simulink model "mcb_pmsm_param_est_f28379d"  (R2024b)
settings: Solver=FixedStepDiscrete  StartTime=0.0  StopTime=12  RelTol=1e-3  EnableMultiTasking=on
InitFcn:
  | mcb_pmsm_param_est_f28379d_data;
values from neighbouring files (symbols this model uses):
  dataType = 'single'    [mcb_pmsm_param_est_f28379d_data.m]
  inverter = evalin('base','inverter')    [mcb_param_est_StopFunc.m]    (also in mcb_pmsm_param_est_f28379d_data.m = mcb_updateInverterParameters(motor,inverter,target))
  target = mcb_SetProcessorDetails('F28379D',PWM_frequency)    [mcb_pmsm_param_est_f28379d_data.m]
  Ts = T_pwm    (= 5e-05)    [mcb_pmsm_param_est_f28379d_data.m]
  Ts_motor = T_pwm/2    (= 2.5e-05)    [mcb_pmsm_param_est_f28379d_data.m]
undefined symbols (not defined in the file or in its folder): Down, GPTRIP1SEL, GPTRIP2SEL, motor, TZ1, TZ2, Up
libraries: simulink x14, c2802xlib x8, c280xlib x5, mcbpmsmparamestlib x5, c2837xDlib x4, mcbpositiondecoderlib x3, svdschedulerlib x2, autolibpmsminterior x2, mcbplantlib x1, mcbcontrolslib x1, svdutilitieslib x1
(part 1 of 3)
settings Model: DataDictionary=mcbEnumerations.sldd  ExtModeTrigDuration=8  Creator=The MathWorks, Inc.  LastModifiedBy=The MathWorks, Inc.
settings SolverCC: AlgebraicLoopSolver=TrustRegion
settings OptimizationCC: DefaultParameterBehavior=Inlined  DefaultUnderspecifiedDataType=single  OptimizeBlockIOStorage=off  ReuseModelBlockBuffer=off  EnhancedBackFolding=on  InitFltsAndDblsToZero=on  NoFixptDivByZeroProtection=on  EfficientFloat2IntCast=on  EfficientMapNaN2IntZero=off  MaxStackSize=1024  OptimizeBlockOrder=speed  DifferentSizesBufferReuse=on  DenormalBehavior=FlushToZero  EfficientTunableParamExpr=on
settings DebuggingCC: MultiTaskDSMMsg=none  ParameterPrecisionLossMsg=none  ParameterTunabilityLossMsg=error  UnconnectedInputMsg=warning  UnconnectedOutputMsg=warning  UnconnectedLineMsg=warning  SubsystemReferenceDiagnosticForUnitTest=warning
settings HardwareCC: ProdBitPerChar=16  ProdBitPerInt=16  ProdBitPerPointer=32  ProdBitPerSizeT=32  ProdBitPerPtrDiffT=32  ProdLargestAtomicInteger=Integer  ProdLargestAtomicFloat=None  ProdWordSize=16  ProdLongLongMode=on  ProdHWDeviceType=Texas Instruments->C2000
settings ModelReferenceCC: EnableRefExpFcnMdlSchedulingChecks=on
settings SFSimCC: MATLABDynamicMemAlloc=off
settings RTWCC: Description=Embedded Coder  SystemTargetFile=ert.tlc  HardwareBoard=TI Delfino F28379D LaunchPad  TemplateMakefile=ert_default_tmf  GenerateReport=on  Toolchain=Texas Instruments Code Composer Studio (C2000)  GPUComputeCapability=3.5  DLArmComputeVersion=19.05
settings CodeAppCC: IgnoreCustomStorageClasses=off  StateflowObjectComments=on
settings ERTTargetCC: CodeReplacementLibrary=TI C28x  ExtModeStaticAllocSize=10000  InlinedParameterPlacement=Hierarchical  ConvertIfToSwitch=off  SuppressUnreachableDefaultCases=off  MemSecPackage=tic2000demospkg  DynamicArrayContainerType=coder::array

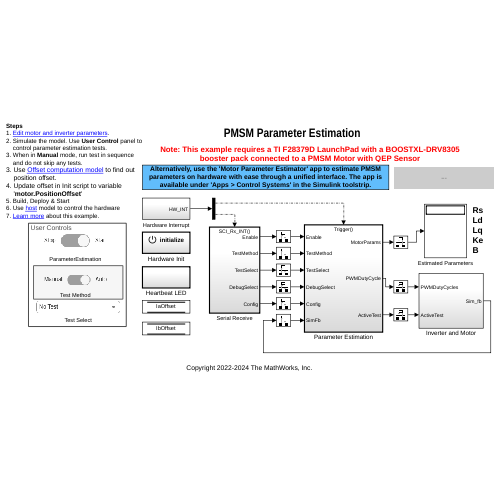
[thumbnail: Simulink's stored preview of the top-level diagram]
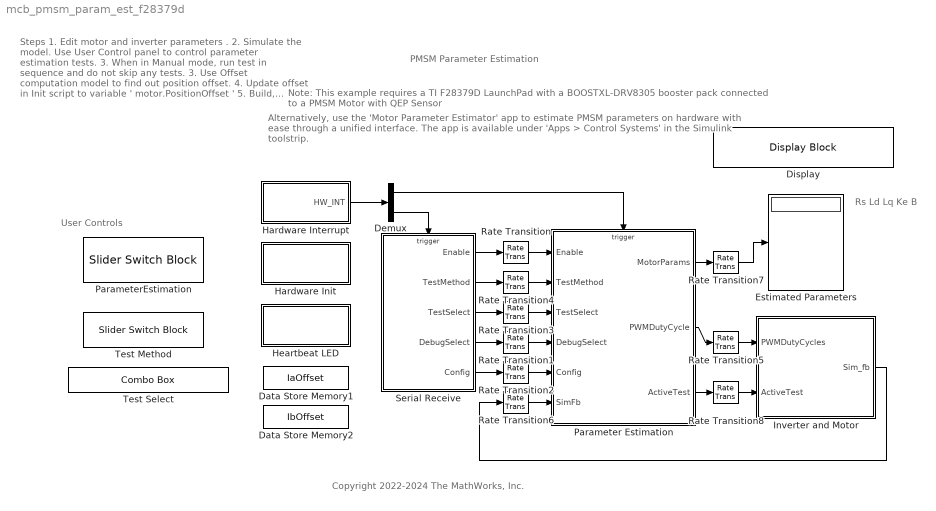
== system mcb_pmsm_param_est_f28379d ==
  note: Alternatively, use the 'Motor Parameter Estimator' app to estimate PMSM parameters on hardware with ease through a unified interface. The app is available under 'Apps > Control Systems' in the Simulink toolstrip.
  note: Note: This example requires a TI F28379D LaunchPad with a BOOSTXL-DRV8305 booster pack connected to a PMSM Motor with QEP Sensor
  note: Copyright 2022-2024 The MathWorks, Inc.
  note: PMSM Parameter Estimation
  note: Rs
      | Ld
      | Lq
      | Ke
      | B
  note: User Controls
  note: Steps
      | 1. Edit motor and inverter parameters .
      | 2. Simulate the model. Use User Control panel to
      | control parameter estimation tests.
      | 3. When in Manual mode, run test in sequence
      | and do not skip any tests.
      | 3. Use Offset computation model to find out
      | position offset.
      | 4. Update offset in Init script to variable
      | ' motor.PositionOffset '
      | 5. Build, Deploy & Start
      | 6. Use host model to control the hardware
      | 7. Learn more about this example.
  Data Store Memory1 : DataStoreMemory  DataStoreName=IaOffset  ReadBeforeWriteMsg=warning  WriteAfterWriteMsg=warning  WriteAfterReadMsg=warning  InitialValue=inverter.CtSensAOffset  ShowAdditionalParam=off
  Data Store Memory2 : DataStoreMemory  DataStoreName=IbOffset  ReadBeforeWriteMsg=warning  WriteAfterWriteMsg=warning  WriteAfterReadMsg=warning  InitialValue=inverter.CtSensBOffset  ShowAdditionalParam=off
  Demux : Demux  Outputs=2
  Display : DisplayBlock  LabelPosition=Hide  Transparency=1
  Estimated Parameters : Display
  Hardware Init : Subsystem  TreatAsAtomicUnit=on
  Hardware Interrupt : Subsystem
  Heartbeat LED : Subsystem  TreatAsAtomicUnit=on
  Inverter and Motor : Subsystem
  Parameter Estimation : Subsystem
  ParameterEstimation : SliderSwitchBlock  LabelPosition=Hide
      settings: Values={{'Stop', 'Start'}, [0 1]}
  Rate Transition{,1..6,8} (8 alike) : RateTransition  Deterministic=off
  Rate Transition7 : RateTransition  Deterministic=off  OutPortSampleTime=0.1
  Serial Receive : Subsystem  SystemSampleTime=1e-3
  Test Method : SliderSwitchBlock  LabelPosition=Hide
      settings: Values={{'Manual', 'Auto'}, [0 1]}
  Test Select : ComboBox  LabelPosition=Hide  SelectedLabel=No Test
      settings: Values={{'No Test', 'Rs', 'Ld', 'Lq', 'Ke, J, B'}, [0 1 2 3 4]}
  wires:
  Demux/1 -> Parameter Estimation/Trigger
  Demux/2 -> Serial Receive/Trigger
  Serial Receive/1(Enable) -> Rate Transition/1
  Rate Transition/1 -> Parameter Estimation/1(Enable)
  Serial Receive/5(Config) -> Rate Transition2/1
  Rate Transition2/1 -> Parameter Estimation/5(Config)
  Serial Receive/3(TestSelect) -> Rate Transition3/1
  Rate Transition3/1 -> Parameter Estimation/3(TestSelect)
  Rate Transition4/1 -> Parameter Estimation/2(TestMethod)
  Serial Receive/2(TestMethod) -> Rate Transition4/1
  Inverter and Motor/1(Sim_fb) -> Rate Transition6/1
  Parameter Estimation/2(PWMDutyCycle) -> Rate Transition5/1
  Rate Transition5/1 -> Inverter and Motor/1(PWMDutyCycles)
  Rate Transition6/1 -> Parameter Estimation/6(SimFb)
  Parameter Estimation/1(MotorParams) -> Rate Transition7/1
  Rate Transition7/1 -> Estimated Parameters/1
  Hardware Interrupt/1(HW_INT) -> Demux/1
  Serial Receive/4(DebugSelect) -> Rate Transition1/1
  Rate Transition1/1 -> Parameter Estimation/4(DebugSelect)
  Parameter Estimation/3(ActiveTest) -> Rate Transition8/1
  Rate Transition8/1 -> Inverter and Motor/2(ActiveTest)

== system mcb_pmsm_param_est_f28379d/Hardware Init ==
  6PWM_Mode : Constant  Priority=1000  Value=0x3A16  OutDataTypeStr=uint16  SampleTime=-1
  ADC_Gain_Setting : Constant  Priority=1000  Value=inverter.SPI_Gain_Setting  OutDataTypeStr=uint16  SampleTime=-1
  Event Listener : EventListener  DisableCoverage=on  EventName=reset
  Mux : Mux  Inputs=2
  Variant Subsystem : Subsystem  Variant=on  VariantControlMode=sim codegen switching
  wires:
  6PWM_Mode/1 -> Mux/1
  ADC_Gain_Setting/1 -> Mux/2
  Mux/1 -> Variant Subsystem/1(In1)

== system mcb_pmsm_param_est_f28379d/Hardware Interrupt ==
  Hardware Interrupt : Subsystem  Variant=on  VariantControlMode=sim codegen switching
  HW_INT : Outport
  wires:
  Hardware Interrupt/1(HW_INT) -> HW_INT/1

== system mcb_pmsm_param_est_f28379d/Heartbeat LED ==
  note: Heartbeat LED 1HZ
  Heartbeat LED : Subsystem  Variant=on  VariantControlMode=sim codegen switching
  RED_LED : Constant  OutDataTypeStr=uint16  SampleTime=0.5
  wires:
  RED_LED/1 -> Heartbeat LED/1(In1)

== system mcb_pmsm_param_est_f28379d/Inverter and Motor ==
  PWMDutyCycles : Inport
  ActiveTest : Inport  Port=2
  Inverter and Motor : Subsystem  Variant=on  VariantControlMode=sim codegen switching
  Sim_fb : Outport  VectorParamsAs1DForOutWhenUnconnected=off
  wires:
  PWMDutyCycles/1 -> Inverter and Motor/1(DutyCycles)
  Inverter and Motor/1(SimFb) -> Sim_fb/1
  ActiveTest/1 -> Inverter and Motor/2(ActiveTest)

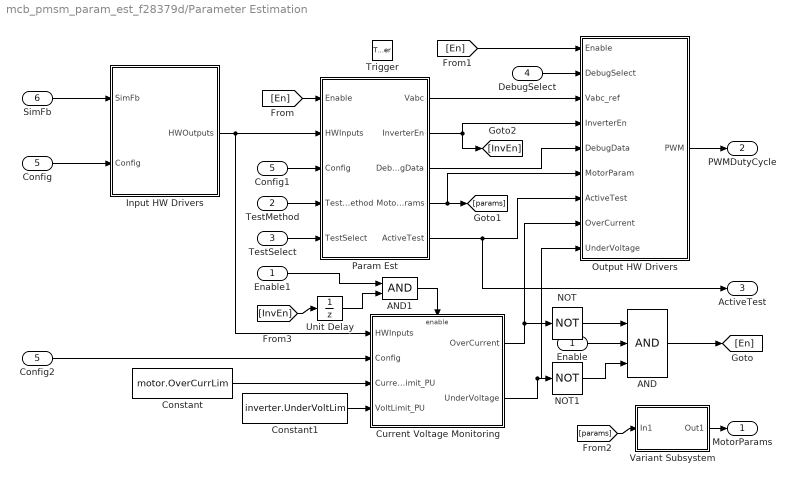
== system mcb_pmsm_param_est_f28379d/Parameter Estimation ==
  Enable : Inport
  TestMethod : Inport  Port=2
  TestSelect : Inport  Port=3
  DebugSelect : Inport  Port=4
  Config : Inport  Port=5
  SimFb : Inport  Port=6
  Trigger : TriggerPort  TriggerType=function-call  VariantControl=Variant  PortDimensions=1
  AND : Logic  Inputs=3  IconShape=distinctive  AllPortsSameDT=off  OutDataTypeStr=boolean
  AND1 : Logic  AllPortsSameDT=off  OutDataTypeStr=boolean
  Config1 : InportShadow  Port=5
  Config2 : InportShadow  Port=5
  Constant : Constant  Value=motor.OverCurrLim  OutDataTypeStr=dataType
  Constant1 : Constant  Value=inverter.UnderVoltLim  OutDataTypeStr=dataType
  Current Voltage Monitoring : Subsystem
  Enable1 : InportShadow
  Input HW Drivers : Subsystem
  NOT : Logic  Operator=NOT  IconShape=distinctive  AllPortsSameDT=off  OutDataTypeStr=boolean
  NOT1 : Logic  Operator=NOT  IconShape=distinctive  AllPortsSameDT=off  OutDataTypeStr=boolean
  Output HW Drivers : Subsystem
  Param Est : Subsystem
  Unit Delay : UnitDelay  SampleTime=-1  HasFrameUpgradeWarning=on
  Variant Subsystem : Subsystem  Variant=on  VariantControlMode=sim codegen switching
  MotorParams : Outport
  PWMDutyCycle : Outport  Port=2
  ActiveTest : Outport  Port=3
  wires:
  Config/1 -> Input HW Drivers/2(Config)
  Param Est/1(Vabc) -> Output HW Drivers/3(Vabc_ref)
  Param Est/2(InverterEn) -> Output HW Drivers/4(InverterEn), [InvEn]
  Param Est/4(MotorParams) -> Output HW Drivers/6(MotorParam), [params]
  Input HW Drivers/1(HWOutputs) -> Param Est/2(HWInputs), Current Voltage Monitoring/1(HWInputs)
  TestSelect/1 -> Param Est/5(TestSelect)
  TestMethod/1 -> Param Est/4(TestMethod)
  SimFb/1 -> Input HW Drivers/1(SimFb)
  Output HW Drivers/1(PWM) -> PWMDutyCycle/1
  Variant Subsystem/1(Out1) -> MotorParams/1
  [En] -> Output HW Drivers/1(Enable)
  Config1/1 -> Param Est/3(Config)
  Config2/1 -> Current Voltage Monitoring/2(Config)
  Param Est/3(DebugData) -> Output HW Drivers/5(DebugData)
  DebugSelect/1 -> Output HW Drivers/2(DebugSelect)
  Constant/1 -> Current Voltage Monitoring/3(CurrentLimit_PU)
  Constant1/1 -> Current Voltage Monitoring/4(VoltLimit_PU)
  Current Voltage Monitoring/1(OverCurrent) -> NOT/1, Output HW Drivers/8(OverCurrent)
  Current Voltage Monitoring/2(UnderVoltage) -> Output HW Drivers/9(UnderVoltage), NOT1/1
  NOT/1 -> AND/1
  NOT1/1 -> AND/3
  Enable/1 -> AND/2
  AND/1 -> [En]
  [En] -> Param Est/1(Enable)
  Param Est/5(ActiveTest) -> ActiveTest/1, Output HW Drivers/7(ActiveTest)
  [params] -> Variant Subsystem/1(In1)
  Unit Delay/1 -> AND1/2
  [InvEn] -> Unit Delay/1
  AND1/1 -> Current Voltage Monitoring/Enable
  Enable1/1 -> AND1/1

== system mcb_pmsm_param_est_f28379d/Serial Receive ==
  SCI_Rx_INT : TriggerPort  TriggerType=function-call  VariantControl=Variant
  Variant Subsystem : Subsystem  Variant=on  VariantControlMode=sim codegen switching
  Enable : Outport
  TestMethod : Outport  Port=2
  TestSelect : Outport  Port=3
  DebugSelect : Outport  Port=4
  Config : Outport  Port=5
  wires:
  Variant Subsystem/1(Enable) -> Enable/1
  Variant Subsystem/2(TestMethod) -> TestMethod/1
  Variant Subsystem/3(TestSelect) -> TestSelect/1
  Variant Subsystem/5(Config) -> Config/1
  Variant Subsystem/4(DebugSelect) -> DebugSelect/1

== system mcb_pmsm_param_est_f28379d/Hardware Init/Variant Subsystem ==
  In1 : Inport
  Code Generation : Subsystem  VariantControl=(codegen)
  Simulation : Subsystem  VariantControl=(sim)

== system mcb_pmsm_param_est_f28379d/Hardware Interrupt/Hardware Interrupt ==
  Codegen : Subsystem  VariantControl=(codegen)
  Sim : Subsystem  VariantControl=(sim)
  HW_INT : Outport  OutputFunctionCall=on

== system mcb_pmsm_param_est_f28379d/Heartbeat LED/Heartbeat LED ==
  In1 : Inport
  Code generation : Subsystem  VariantControl=(codegen)
  Simulation : Subsystem  VariantControl=(sim)

== system mcb_pmsm_param_est_f28379d/Inverter and Motor/Inverter and Motor ==
  DutyCycles : Inport
  ActiveTest : Inport  Port=2
  Codegeneration : Subsystem  VariantControl=(codegen)
  Sim : Subsystem  VariantControl=(sim)
  SimFb : Outport  VectorParamsAs1DForOutWhenUnconnected=off

== system mcb_pmsm_param_est_f28379d/Parameter Estimation/Current Voltage Monitoring ==
  HWInputs : Inport
  Config : Inport  Port=2
  CurrentLimit_PU : Inport  Port=3
  VoltLimit_PU : Inport  Port=4
  Enable : EnablePort  StatesWhenEnabling=reset
  Current and Voltage Monitoring : Subsystem
  NOR : Logic  Operator=NOR  IconShape=distinctive  AllPortsSameDT=off  OutDataTypeStr=boolean
  Unit Delay : UnitDelay  SampleTime=-1  HasFrameUpgradeWarning=on
  OverCurrent : Outport  InitialOutput=0
  UnderVoltage : Outport  Port=2  InitialOutput=0
  wires:
  HWInputs/1 -> Current and Voltage Monitoring/1(HWInputs)
  Current and Voltage Monitoring/2(UnderVoltage) -> UnderVoltage/1, NOR/2
  VoltLimit_PU/1 -> Current and Voltage Monitoring/4(VoltLimit)
  NOR/1 -> Unit Delay/1
  CurrentLimit_PU/1 -> Current and Voltage Monitoring/3(CurrentLimit)
  Current and Voltage Monitoring/1(OverCurrent) -> NOR/1, OverCurrent/1
  Unit Delay/1 -> Current and Voltage Monitoring/Enable
  Config/1 -> Current and Voltage Monitoring/2(Config)

== system mcb_pmsm_param_est_f28379d/Parameter Estimation/Input HW Drivers ==
  SimFb : Inport
  Config : Inport  Port=2
  Bus Creator : BusCreator  Inputs=5
  Demux : Demux  Outputs=2
  Input Scaling : Subsystem
  Variant Subsystem : Subsystem  Variant=on  VariantControlMode=sim codegen switching
  HWOutputs : Outport
  wires:
  Config/1 -> Input Scaling/5(Config)
  Bus Creator/1 -> HWOutputs/1
  Input Scaling/1(Iabc) -> Bus Creator/1  "Iabc"
  Input Scaling/2(Vdc) -> Bus Creator/2  "Vdc"
  Input Scaling/5(EnClosedLoop) -> Bus Creator/5  "EnClosedLoop"
  Input Scaling/4(Pos_PU) -> Bus Creator/4  "Theta"
  Input Scaling/3(Speed_RPM) -> Bus Creator/3  "Speed"
  SimFb/1 -> Variant Subsystem/1(SimFb)
  Variant Subsystem/1(IabADC) -> Input Scaling/1(Iab_ADC)
  Variant Subsystem/2(VdcADC) -> Input Scaling/2(Vdc_ADC)
  Variant Subsystem/3(eQEP) -> Demux/1
  Demux/1 -> Input Scaling/3(QEPPositionCount)
  Demux/2 -> Input Scaling/4(QEPIndexLatch)

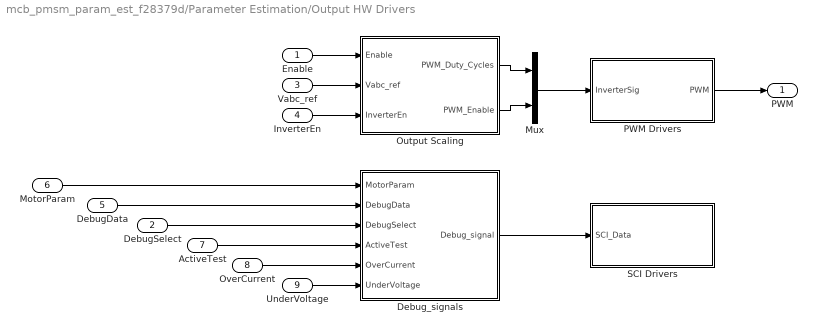
== system mcb_pmsm_param_est_f28379d/Parameter Estimation/Output HW Drivers ==
  Enable : Inport
  DebugSelect : Inport  Port=2
  Vabc_ref : Inport  Port=3
  InverterEn : Inport  Port=4
  DebugData : Inport  Port=5
  MotorParam : Inport  Port=6
  ActiveTest : Inport  Port=7
  OverCurrent : Inport  Port=8
  UnderVoltage : Inport  Port=9
  Debug_signals : Subsystem
  Mux : Mux  Inputs=2
  Output Scaling : Subsystem
  PWM Drivers : Subsystem  Variant=on  VariantControlMode=sim codegen switching
  SCI Drivers : Subsystem  Variant=on  VariantControlMode=sim codegen switching
  PWM : Outport
  wires:
  Output Scaling/2(PWM_Enable) -> Mux/2
  Mux/1 -> PWM Drivers/1(InverterSig)
  InverterEn/1 -> Output Scaling/3(InverterEn)
  MotorParam/1 -> Debug_signals/1(MotorParam)
  Vabc_ref/1 -> Output Scaling/2(Vabc_ref)
  Output Scaling/1(PWM_Duty_Cycles) -> Mux/1
  Enable/1 -> Output Scaling/1(Enable)
  Debug_signals/1(Debug_signal) -> SCI Drivers/1(SCI_Data)
  PWM Drivers/1(PWM) -> PWM/1
  DebugData/1 -> Debug_signals/2(DebugData)
  DebugSelect/1 -> Debug_signals/3(DebugSelect)
  OverCurrent/1 -> Debug_signals/5(OverCurrent)
  UnderVoltage/1 -> Debug_signals/6(UnderVoltage)
  ActiveTest/1 -> Debug_signals/4(ActiveTest)

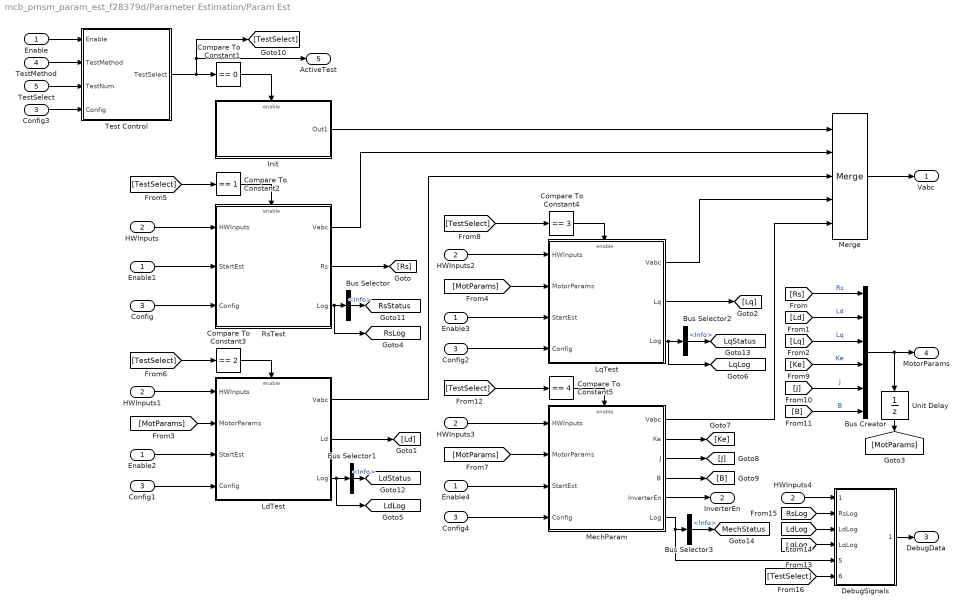
== system mcb_pmsm_param_est_f28379d/Parameter Estimation/Param Est ==
  Enable : Inport
  HWInputs : Inport  Port=2
  Config : Inport  Port=3
  TestMethod : Inport  Port=4
  TestSelect : Inport  Port=5
  Bus Creator : BusCreator  Inputs=6
  Bus Selector{,1..3} (4 alike) : BusSelector  OutputSignals=Info
  Compare To Constant1 : simulink/Logic and Bit Operations/Compare To Constant  relop===  const=0  OutDataTypeStr=boolean
  Compare To Constant2 : simulink/Logic and Bit Operations/Compare To Constant  relop===  const=1  OutDataTypeStr=boolean
  Compare To Constant3 : simulink/Logic and Bit Operations/Compare To Constant  relop===  const=2  OutDataTypeStr=boolean
  Compare To Constant4 : simulink/Logic and Bit Operations/Compare To Constant  relop===  const=3  OutDataTypeStr=boolean
  Compare To Constant5 : simulink/Logic and Bit Operations/Compare To Constant  relop===  const=4  OutDataTypeStr=boolean
  Config{1..4} (4 alike) : InportShadow  Port=3
  DebugSignals : Subsystem
  Enable{1..4} (4 alike) : InportShadow
  HWInputs{1..4} (4 alike) : InportShadow  Port=2
  Init : Subsystem
  LdTest : Subsystem
  LqTest : Subsystem
  MechParam : Subsystem
  Merge : Merge  Inputs=5
  RsTest : Subsystem
  Test Control : Subsystem
  Unit Delay : UnitDelay  SampleTime=-1  HasFrameUpgradeWarning=on
  Vabc : Outport
  InverterEn : Outport  Port=2
  DebugData : Outport  Port=3
  MotorParams : Outport  Port=4
  ActiveTest : Outport  Port=5
  tag scope: LdLog=global, LdStatus=global, LqLog=global, LqStatus=global, MechStatus=global, RsLog=global, RsStatus=global
  wires:
  Config/1 -> RsTest/3(Config)
  Config1/1 -> LdTest/4(Config)
  Config2/1 -> LqTest/4(Config)
  HWInputs/1 -> RsTest/1(HWInputs)
  HWInputs1/1 -> LdTest/1(HWInputs)
  HWInputs2/1 -> LqTest/1(HWInputs)
  Bus Creator/1 -> MotorParams/1, Unit Delay/1
  RsTest/2(Rs) -> [Rs]
  LdTest/3(Log) -> [LdLog], Bus Selector1/1
  LdTest/2(Ld) -> [Ld]
  LqTest/2(Lq) -> [Lq]
  LqTest/3(Log) -> [LqLog], Bus Selector2/1
  [Rs] -> Bus Creator/1  "Rs"
  [Ld] -> Bus Creator/2  "Ld"
  [Lq] -> Bus Creator/3  "Lq"
  Unit Delay/1 -> [MotParams]
  [MotParams] -> LdTest/2(MotorParams)
  [MotParams] -> LqTest/2(MotorParams)
  Test Control/1(TestSelect) -> [TestSelect], ActiveTest/1, Compare To Constant1/1
  Compare To Constant1/1 -> Init/Enable
  Compare To Constant2/1 -> RsTest/Enable
  Compare To Constant3/1 -> LdTest/Enable
  Compare To Constant4/1 -> LqTest/Enable
  Bus Selector1/1 -> [LdStatus]  "<Info>"
  Bus Selector2/1 -> [LqStatus]  "<Info>"
  Compare To Constant5/1 -> MechParam/Enable
  HWInputs3/1 -> MechParam/1(HWInputs)
  Config4/1 -> MechParam/4(Config)
  [MotParams] -> MechParam/2(MotorParams)
  MechParam/6(Log) -> DebugSignals/5(MechLog), Bus Selector3/1
  MechParam/2(Ke) -> [Ke]
  [Ke] -> Bus Creator/4  "Ke"
  Merge/1 -> Vabc/1
  Init/1(Out1) -> Merge/1
  RsTest/1(Vabc) -> Merge/2
  LdTest/1(Vabc) -> Merge/3
  LqTest/1(Vabc) -> Merge/4
  MechParam/1(Vabc) -> Merge/5
  MechParam/3(J) -> [J]
  MechParam/4(B) -> [B]
  [J] -> Bus Creator/5  "J"
  [B] -> Bus Creator/6  "B"
  MechParam/5(InverterEn) -> InverterEn/1
  Enable/1 -> Test Control/1(Enable)
  TestSelect/1 -> Test Control/3(TestNum)
  TestMethod/1 -> Test Control/2(TestMethod)
  [TestSelect] -> Compare To Constant2/1
  [TestSelect] -> Compare To Constant3/1
  [TestSelect] -> Compare To Constant4/1
  [TestSelect] -> Compare To Constant5/1
  Enable1/1 -> RsTest/2(StartEst)
  Enable2/1 -> LdTest/3(StartEst)
  Enable3/1 -> LqTest/3(StartEst)
  Enable4/1 -> MechParam/3(StartEst)
  Bus Selector/1 -> [RsStatus]  "<Info>"
  Bus Selector3/1 -> [MechStatus]  "<Info>"
  HWInputs4/1 -> DebugSignals/1(HWInpust)
  RsTest/3(Log) -> [RsLog], Bus Selector/1
  [LqLog] -> DebugSignals/4(LqLog)
  [LdLog] -> DebugSignals/3(LdLog)
  [RsLog] -> DebugSignals/2(RsLog)
  DebugSignals/1(DebugData) -> DebugData/1
  Config3/1 -> Test Control/4(Config)
  [TestSelect] -> DebugSignals/6(ActiveTest)

== system mcb_pmsm_param_est_f28379d/Parameter Estimation/Variant Subsystem ==
  In1 : Inport
  Codegen : Subsystem  VariantControl=(codegen)
  Sim : Subsystem  VariantControl=(sim)
  Out1 : Outport

== system mcb_pmsm_param_est_f28379d/Serial Receive/Variant Subsystem ==
  Codegen : Subsystem  VariantControl=(codegen)
  Sim : Subsystem  VariantControl=(sim)
  Enable : Outport
  TestMethod : Outport  Port=2
  TestSelect : Outport  Port=3
  DebugSelect : Outport  Port=4
  Config : Outport  Port=5

== system mcb_pmsm_param_est_f28379d/Hardware Init/Variant Subsystem/Code Generation ==
  note: for BoostXL-DRV8305 connected to LaunchXL-28379D
  note: System Outputs
  note: Enable ADC offset calibration only when motor is not loaded and not rotating due to external factors
  In1 : Inport
  ADC Calib Enable : Constant  Value=inverter.ADCOffsetCalibEnable  OutDataTypeStr=Inherit: Inherit via back propagation
  "Calculate ADC Offset " : Subsystem  Priority=1001  TreatAsAtomicUnit=on
  DRV Enable : Subsystem  Priority=1
  Default ADC Offset : Subsystem  Priority=1001  TreatAsAtomicUnit=on
  NOT : Logic  Operator=NOT  IconShape=distinctive  AllPortsSameDT=off  OutDataTypeStr=boolean
  wires:
  In1/1 -> DRV Enable/1(In)
  NOT/1 -> Default ADC Offset/Enable
  ADC Calib Enable/1 -> NOT/1, "Calculate ADC Offset "/Enable

== system mcb_pmsm_param_est_f28379d/Hardware Init/Variant Subsystem/Simulation ==
  In1 : Inport
  Constant : Constant  Value=inverter.CtSensAOffset  OutDataTypeStr=Inherit: Inherit via back propagation
  Constant1 : Constant  Value=inverter.CtSensBOffset  OutDataTypeStr=Inherit: Inherit via back propagation
  Data Store Write1 : DataStoreWrite  DataStoreName=IaOffset  IndexOptions=Index vector (dialog)  Indices=1  OutputSizes=1
  Data Store Write2 : DataStoreWrite  DataStoreName=IbOffset  IndexOptions=Index vector (dialog)  Indices=1  OutputSizes=1
  Terminator : Terminator
  wires:
  In1/1 -> Terminator/1
  Constant/1 -> Data Store Write1/1
  Constant1/1 -> Data Store Write2/1

== system mcb_pmsm_param_est_f28379d/Hardware Interrupt/Hardware Interrupt/Codegen ==
  HWI_ADCB1_INT : svdschedulerlib/Hardware Interrupt v2  ISRGroup=ADC - Analog to Digital Converter  ISRName=ADCA1_INT  ISRNumber=32  NumEventsToServe=1  EventsList=[{'on','EOC event','1'};{'off','Overflow event','2'};{'off','Custom event','3'};{'off','Default event','4'}]  SelectedEvents={'event1'}  TaskPriority=30  DisablePreemption=off  ClearInterruptFlagsAtEndOfEvent=on  InterruptDefinitionFile=$(TARGET_ROOT)/registry/interrupts/F2837xS_interrupts.xml  HardwareBoard=F2837x  EnableSimPort=off
      settings: LibrarySourceBlock=c2000lib/Scheduling/Hardware Interrupt
  HWI_SCIA_RX_INT : svdschedulerlib/Hardware Interrupt v2  ISRGroup=ADC - Analog to Digital Converter  ISRName=ADCA1_INT  ISRNumber=32  NumEventsToServe=1  EventsList=[{'on','EOC event','1'};{'off','Overflow event','2'};{'off','Custom event','3'};{'off','Default event','4'}]  SelectedEvents={'event1'}  TaskPriority=50  DisablePreemption=on  ClearInterruptFlagsAtEndOfEvent=on  InterruptDefinitionFile=$(TARGET_ROOT)/registry/interrupts/F2837xS_interrupts.xml  HardwareBoard=F2837x  EnableSimPort=off
      settings: LibrarySourceBlock=c2000lib/Scheduling/Hardware Interrupt
  Mux : Mux  Inputs=2
  HW_INT : Outport
  wires:
  Mux/1 -> HW_INT/1
  HWI_ADCB1_INT/1 -> Mux/1
  HWI_SCIA_RX_INT/1 -> Mux/2

== system mcb_pmsm_param_est_f28379d/Hardware Interrupt/Hardware Interrupt/Sim ==
  ADCINT1 : simulink/Ports & Subsystems/Function-Call Generator  sample_time=Ts  numberOfIterations=1  DisallowWideOutput=off
  Mux : Mux  Inputs=2
  SCI_Rx_INT : simulink/Ports & Subsystems/Function-Call Generator  sample_time=0.1  numberOfIterations=1  DisallowWideOutput=off
  HW_INT : Outport
  wires:
  ADCINT1/1 -> Mux/1
  SCI_Rx_INT/1 -> Mux/2
  Mux/1 -> HW_INT/1

== system mcb_pmsm_param_est_f28379d/Heartbeat LED/Heartbeat LED/Code generation ==
  In1 : Inport
  Digital Output : c2837xDlib/Digital Output  GPIO_Number=GPIO32~GPIO39  GPIO_Bit0=off  GPIO_BIT0_Toggle=on  GPIO_Bit1=off  GPIO_BIT1_Toggle=off  GPIO_Bit2=on  GPIO_BIT2_Toggle=on  GPIO_Bit3=off  GPIO_BIT3_Toggle=off  GPIO_Bit4=off  GPIO_BIT4_Toggle=off  GPIO_Bit5=off  GPIO_BIT5_Toggle=off  GPIO_Bit6=off  GPIO_BIT6_Toggle=off  GPIO_Bit7=off  GPIO_BIT7_Toggle=off
  wires:
  In1/1 -> Digital Output/1

== system mcb_pmsm_param_est_f28379d/Heartbeat LED/Heartbeat LED/Simulation ==
  In1 : Inport
  Simulation_Terminator : Terminator
  wires:
  In1/1 -> Simulation_Terminator/1

== system mcb_pmsm_param_est_f28379d/Inverter and Motor/Inverter and Motor/Codegeneration ==
  DutyCycles : Inport
  ActiveTest : Inport  Port=2
  Ground : Ground
  Terminator : Terminator
  Terminator1 : Terminator
  SimFb : Outport  VectorParamsAs1DForOutWhenUnconnected=off
  wires:
  DutyCycles/1 -> Terminator/1
  Ground/1 -> SimFb/1
  ActiveTest/1 -> Terminator1/1

== system mcb_pmsm_param_est_f28379d/Inverter and Motor/Inverter and Motor/Sim ==
  DutyCycles : Inport
  ActiveTest : Inport  Port=2
  Inverter : Subsystem
  Motor : Subsystem
  RT1 : RateTransition  Deterministic=off  OutPortSampleTime=Ts_simulink
  RT3 : RateTransition  Deterministic=off  OutPortSampleTime=Ts_simulink
  Rate Transition : RateTransition  Deterministic=off  OutPortSampleTime=Ts_motor
  Sensor_Measurements : Subsystem
  SimFb : Outport  VectorParamsAs1DForOutWhenUnconnected=off
  wires:
  Sensor_Measurements/1(Sim_fb) -> SimFb/1
  DutyCycles/1 -> Inverter/1(Duty_abc)
  Inverter/1(Vabc) -> Rate Transition/1
  RT3/1 -> Sensor_Measurements/1(Info)
  RT1/1 -> Sensor_Measurements/2(PhaseCurr)
  Rate Transition/1 -> Motor/1(PhaseVolt)
  Motor/1(Info) -> RT3/1
  Motor/2(Iabc) -> RT1/1
  ActiveTest/1 -> Motor/2(ActiveTest)

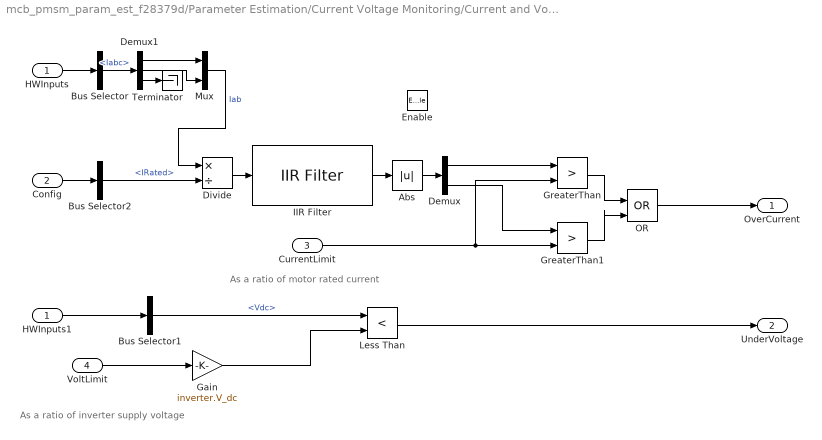
== system mcb_pmsm_param_est_f28379d/Parameter Estimation/Current Voltage Monitoring/Current and Voltage Monitoring ==
  note: As a ratio of motor rated current
  note: As a ratio of inverter supply voltage
  HWInputs : Inport
  Config : Inport  Port=2
  CurrentLimit : Inport  Port=3
  VoltLimit : Inport  Port=4
  Enable : EnablePort
  Abs : Abs  SaturateOnIntegerOverflow=off
  Bus Selector : BusSelector  OutputSignals=Iabc
  Bus Selector1 : BusSelector  OutputSignals=Vdc
  Bus Selector2 : BusSelector  OutputSignals=IRated
  Demux : Demux  Outputs=2
  Demux1 : Demux  Outputs=3
  Divide : Product  Inputs=*/  RndMeth=Simplest  OutDataTypeStr=Inherit: Same as first input
  Gain : Gain  Gain=inverter.V_dc  RndMeth=Simplest  OutDataTypeStr=Inherit: Same as input
  GreaterThan : RelationalOperator  Operator=>  OutDataTypeStr=boolean  RndMeth=Simplest  InputSameDT=off
  GreaterThan1 : RelationalOperator  Operator=>  OutDataTypeStr=boolean  RndMeth=Simplest  InputSameDT=off
  HWInputs1 : InportShadow
  IIR Filter : mcbcontrolslib/IIR Filter  VariantControl=Low Pass Filter  VariantSelect=Low-pass  FilterConstantInputType=Specify via dialog  Filter_constant=0.01  advancedSettings=off  Ts=50e-6  cutOff_freq=32.1525
      settings: LibrarySourceBlock=mcbhdllib/Signal Management/IIR Filter
  Less Than : RelationalOperator  Operator=<  OutDataTypeStr=boolean  RndMeth=Simplest  InputSameDT=off
  Mux : Mux  Inputs=2
  OR : Logic  Operator=OR  IconShape=distinctive  AllPortsSameDT=off  OutDataTypeStr=boolean
  Terminator : Terminator
  OverCurrent : Outport
  UnderVoltage : Outport  Port=2
  wires:
  Less Than/1 -> UnderVoltage/1
  GreaterThan1/1 -> OR/2
  Mux/1 -> Divide/1  "Iab"
  GreaterThan/1 -> OR/1
  CurrentLimit/1 -> GreaterThan1/2, GreaterThan/2
  Demux/2 -> GreaterThan1/1
  OR/1 -> OverCurrent/1
  Abs/1 -> Demux/1
  Divide/1 -> IIR Filter/1
  VoltLimit/1 -> Gain/1
  IIR Filter/1 -> Abs/1
  Demux/1 -> GreaterThan/1
  HWInputs/1 -> Bus Selector/1
  Bus Selector/1 -> Demux1/1  "<Iabc>"
  Demux1/1 -> Mux/1
  Demux1/2 -> Mux/2
  Demux1/3 -> Terminator/1
  HWInputs1/1 -> Bus Selector1/1
  Bus Selector1/1 -> Less Than/1  "<Vdc>"
  Config/1 -> Bus Selector2/1
  Bus Selector2/1 -> Divide/2  "<IRated>"
  Gain/1 -> Less Than/2

== system mcb_pmsm_param_est_f28379d/Parameter Estimation/Input HW Drivers/Input Scaling ==
  Iab_ADC : Inport
  Vdc_ADC : Inport  Port=2
  QEPPositionCount : Inport  Port=3
  QEPIndexLatch : Inport  Port=4
  Config : Inport  Port=5
  " Calculate Position and Speed" : Subsystem
  Calculate Phase Currents : Subsystem
  Subsystem : Subsystem
  Iabc : Outport
  Vdc : Outport  Port=2
  Speed_RPM : Outport  Port=3
  Pos_PU : Outport  Port=4
  EnClosedLoop : Outport  Port=5
  wires:
  " Calculate Position and Speed"/2(Speed_RPM) -> Speed_RPM/1
  Calculate Phase Currents/1(Iabc) -> Iabc/1
  QEPPositionCount/1 -> " Calculate Position and Speed"/1(QEPPositionCount)
  " Calculate Position and Speed"/1(Theta_e) -> Pos_PU/1
  Iab_ADC/1 -> Calculate Phase Currents/1(Iab_ADC)
  QEPIndexLatch/1 -> " Calculate Position and Speed"/2(QEPIndexLatch)
  Config/1 -> Calculate Phase Currents/2(Config), Subsystem/1(Config)
  " Calculate Position and Speed"/3(IndexFound) -> EnClosedLoop/1
  Vdc_ADC/1 -> Subsystem/2(Vdc_ADC)
  Subsystem/1(Vdc) -> Vdc/1

== system mcb_pmsm_param_est_f28379d/Parameter Estimation/Input HW Drivers/Variant Subsystem ==
  SimFb : Inport
  Sim : Subsystem  VariantControl=(sim)
  codegen : Subsystem  VariantControl=(codegen)
  IabADC : Outport
  VdcADC : Outport  Port=2
  eQEP : Outport  Port=3

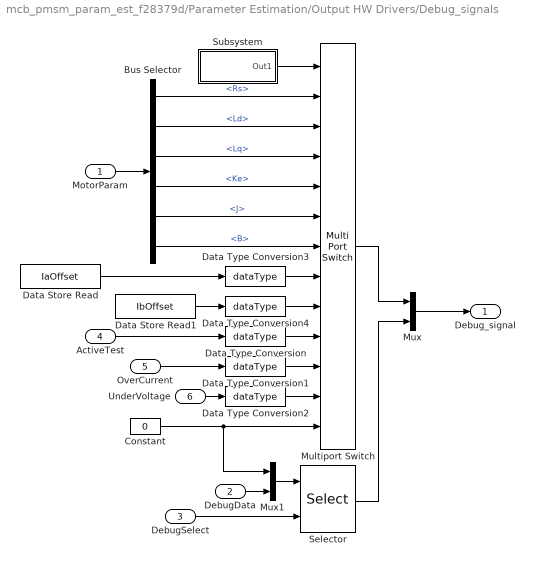
== system mcb_pmsm_param_est_f28379d/Parameter Estimation/Output HW Drivers/Debug_signals ==
  MotorParam : Inport
  DebugData : Inport  Port=2
  DebugSelect : Inport  Port=3
  ActiveTest : Inport  Port=4
  OverCurrent : Inport  Port=5
  UnderVoltage : Inport  Port=6
  Bus Selector : BusSelector  OutputSignals=Rs,Ld,Lq,Ke,J,B
  Constant : Constant  Value=0  OutDataTypeStr=dataType
  Data Store Read : DataStoreRead  DataStoreName=IaOffset  IndexOptions=Index vector (dialog)  Indices=1  OutputSizes=1
  Data Store Read1 : DataStoreRead  DataStoreName=IbOffset  IndexOptions=Index vector (dialog)  Indices=1  OutputSizes=1
  Data Type Conversion{,1..4} (5 alike) : DataTypeConversion  OutDataTypeStr=dataType  RndMeth=Simplest  SaturateOnIntegerOverflow=off
  Multiport Switch : MultiPortSwitch  Inputs=12  DiagnosticForDefault=Warning  OutDataTypeStr=dataType  RndMeth=Simplest  SaturateOnIntegerOverflow=off  InputSameDT=off
  Mux : Mux  Inputs=2
  Mux1 : Mux  Inputs=2
  Selector : Selector  IndexMode=Zero-based  InputPortWidth=13  IndexOptions=Index vector (port)  Indices=[1 3]  OutputSizes=1
  Subsystem : Subsystem
  Debug_signal : Outport
  wires:
  Multiport Switch/1 -> Mux/1
  Subsystem/1(Out1) -> Multiport Switch/1
  MotorParam/1 -> Bus Selector/1
  Mux/1 -> Debug_signal/1
  Bus Selector/1 -> Multiport Switch/2  "<Rs>"
  Bus Selector/2 -> Multiport Switch/3  "<Ld>"
  Bus Selector/3 -> Multiport Switch/4  "<Lq>"
  Bus Selector/4 -> Multiport Switch/5  "<Ke>"
  Bus Selector/5 -> Multiport Switch/6  "<J>"
  Bus Selector/6 -> Multiport Switch/7  "<B>"
  Selector/1 -> Mux/2
  DebugSelect/1 -> Selector/2
  ActiveTest/1 -> Data Type Conversion/1
  OverCurrent/1 -> Data Type Conversion1/1
  UnderVoltage/1 -> Data Type Conversion2/1
  Constant/1 -> Mux1/1, Multiport Switch/13
  Data Type Conversion3/1 -> Multiport Switch/8
  Data Type Conversion4/1 -> Multiport Switch/9
  Data Type Conversion/1 -> Multiport Switch/10
  Data Type Conversion1/1 -> Multiport Switch/11
  Data Type Conversion2/1 -> Multiport Switch/12
  Data Store Read/1 -> Data Type Conversion3/1
  Data Store Read1/1 -> Data Type Conversion4/1
  Mux1/1 -> Selector/1
  DebugData/1 -> Mux1/2

== system mcb_pmsm_param_est_f28379d/Parameter Estimation/Output HW Drivers/Output Scaling ==
  Enable : Inport
  Vabc_ref : Inport  Port=2
  InverterEn : Inport  Port=3
  AND : Logic  IconShape=distinctive  AllPortsSameDT=off  OutDataTypeStr=boolean
  Constant : Constant  Value=0.5  OutDataTypeStr=dataType  SampleTime=-1
  Data Type Conversion : DataTypeConversion  OutDataTypeStr=dataType  SaturateOnIntegerOverflow=off  RndMeth=Floor
  One_by_Two : Gain  Gain=0.5  RndMeth=Simplest  OutDataTypeStr=Inherit: Same as input
  Sum : Sum  Inputs=|++
  PWM_Duty_Cycles : Outport
  PWM_Enable : Outport  Port=2
  wires:
  Constant/1 -> Sum/2
  Vabc_ref/1 -> One_by_Two/1
  Sum/1 -> PWM_Duty_Cycles/1
  Enable/1 -> AND/2
  One_by_Two/1 -> Sum/1
  Data Type Conversion/1 -> PWM_Enable/1
  InverterEn/1 -> AND/1
  AND/1 -> Data Type Conversion/1

== system mcb_pmsm_param_est_f28379d/Parameter Estimation/Output HW Drivers/PWM Drivers ==
  InverterSig : Inport
  Codegen : Subsystem  VariantControl=(codegen)
  Sim : Subsystem  VariantControl=(sim)
  PWM : Outport

== system mcb_pmsm_param_est_f28379d/Parameter Estimation/Output HW Drivers/SCI Drivers ==
  SCI_Data : Inport
  Codegen : Subsystem  VariantControl=(codegen)
  Sim : Subsystem  VariantControl=(sim)

== system mcb_pmsm_param_est_f28379d/Parameter Estimation/Param Est/DebugSignals ==
  HWInpust : Inport
  RsLog : Inport  Port=2
  LdLog : Inport  Port=3
  LqLog : Inport  Port=4
  MechLog : Inport  Port=5
  ActiveTest : Inport  Port=6
  Bus Selector : BusSelector  OutputSignals=Iabc,Vdc,Speed,Theta
  Demux : Demux  Outputs=2
  Mux : Mux  Inputs=12
  Selector : Selector  InputPortWidth=3  IndexOptions=Index vector (dialog)  Indices=[1 2]  OutputSizes=1
  Subsystem : Subsystem
  Terminator1 : Terminator
  DebugData : Outport
  wires:
  Mux/1 -> DebugData/1
  HWInpust/1 -> Bus Selector/1
  Demux/1 -> Mux/1
  Demux/2 -> Mux/2
  Bus Selector/2 -> Mux/3  "<Vdc>"
  Bus Selector/3 -> Mux/4  "<Speed>"
  Bus Selector/4 -> Mux/5  "<Theta>"
  RsLog/1 -> Terminator1/1
  LdLog/1 -> Subsystem/2(LdLog)
  LqLog/1 -> Subsystem/3(LqLog)
  MechLog/1 -> Subsystem/4(MechLog)
  ActiveTest/1 -> Subsystem/1(ActoveTest)
  Subsystem/7(CoastDownTime) -> Mux/12
  Subsystem/5(InjFreq) -> Mux/10
  Subsystem/4(Vq) -> Mux/9
  Subsystem/6(PhaseDiff) -> Mux/11
  Subsystem/3(Vd) -> Mux/8
  Subsystem/2(Iq) -> Mux/7
  Subsystem/1(Id) -> Mux/6
  Bus Selector/1 -> Selector/1  "<Iabc>"
  Selector/1 -> Demux/1

== system mcb_pmsm_param_est_f28379d/Parameter Estimation/Param Est/Init ==
  Enable : EnablePort
  Constant : Constant  Value=[0 0 0]  OutDataTypeStr=dataType
  Out1 : Outport  InitialOutput=[0 0 0]
  wires:
  Constant/1 -> Out1/1

== system mcb_pmsm_param_est_f28379d/Parameter Estimation/Param Est/LdTest ==
  HWInputs : Inport
  MotorParams : Inport  Port=2
  StartEst : Inport  Port=3
  Config : Inport  Port=4
  Enable : EnablePort  StatesWhenEnabling=reset
  Bus Selector : BusSelector  OutputSignals=Iabc
  Bus Selector1 : BusSelector  OutputSignals=Rs
  Ld Estimator : mcbpmsmparamestlib/Ld Estimator
  Vabc : Outport
  Ld : Outport  Port=2
  Log : Outport  Port=3
  wires:
  Config/1 -> Ld Estimator/4
  MotorParams/1 -> Bus Selector1/1
  HWInputs/1 -> Bus Selector/1
  Bus Selector1/1 -> Ld Estimator/2  "<Rs>"
  Bus Selector/1 -> Ld Estimator/1  "<Iabc>"
  Ld Estimator/3 -> Log/1
  Ld Estimator/2 -> Ld/1
  Ld Estimator/1 -> Vabc/1
  StartEst/1 -> Ld Estimator/3

== system mcb_pmsm_param_est_f28379d/Parameter Estimation/Param Est/LqTest ==
  HWInputs : Inport
  MotorParams : Inport  Port=2
  StartEst : Inport  Port=3
  Config : Inport  Port=4
  Enable : EnablePort  StatesWhenEnabling=reset
  Bus Selector : BusSelector  OutputSignals=Iabc
  Bus Selector1 : BusSelector  OutputSignals=Rs
  Lq Estimator : mcbpmsmparamestlib/Lq Estimator
  Vabc : Outport
  Lq : Outport  Port=2
  Log : Outport  Port=3
  wires:
  Lq Estimator/1 -> Vabc/1
  HWInputs/1 -> Bus Selector/1
  MotorParams/1 -> Bus Selector1/1
  Lq Estimator/2 -> Lq/1
  Lq Estimator/3 -> Log/1
  Config/1 -> Lq Estimator/4
  Bus Selector1/1 -> Lq Estimator/2  "<Rs>"
  Bus Selector/1 -> Lq Estimator/1  "<Iabc>"
  StartEst/1 -> Lq Estimator/3

== system mcb_pmsm_param_est_f28379d/Parameter Estimation/Param Est/MechParam ==
  HWInputs : Inport
  MotorParams : Inport  Port=2
  StartEst : Inport  Port=3
  Config : Inport  Port=4
  Enable : EnablePort  StatesWhenEnabling=reset
  Bus Selector : BusSelector  OutputSignals=Rs,Ld
  Bus Selector3 : BusSelector  OutputSignals=Iabc,Vdc,Theta,Speed,EnClosedLoop
  Mechanical Parameter Estimator : mcbpmsmparamestlib/Mechanical Parameter Estimator
  Vabc : Outport
  Ke : Outport  Port=2
  J : Outport  Port=3
  B : Outport  Port=4
  InverterEn : Outport  Port=5  OutputWhenDisabled=reset  InitialOutput=1
  Log : Outport  Port=6
  wires:
  Bus Selector/1 -> Mechanical Parameter Estimator/5  "<Rs>"
  MotorParams/1 -> Bus Selector/1
  Config/1 -> Mechanical Parameter Estimator/9
  Bus Selector/2 -> Mechanical Parameter Estimator/6  "<Ld>"
  Mechanical Parameter Estimator/3 -> J/1
  Mechanical Parameter Estimator/2 -> Ke/1
  Mechanical Parameter Estimator/4 -> B/1
  Mechanical Parameter Estimator/1 -> Vabc/1
  HWInputs/1 -> Bus Selector3/1
  Bus Selector3/1 -> Mechanical Parameter Estimator/1  "<Iabc>"
  Bus Selector3/2 -> Mechanical Parameter Estimator/2  "<Vdc>"
  Mechanical Parameter Estimator/6 -> Log/1
  Mechanical Parameter Estimator/5 -> InverterEn/1
  Bus Selector3/5 -> Mechanical Parameter Estimator/7  "<EnClosedLoop>"
  StartEst/1 -> Mechanical Parameter Estimator/8
  Bus Selector3/3 -> Mechanical Parameter Estimator/3  "<Theta>"
  Bus Selector3/4 -> Mechanical Parameter Estimator/4  "<Speed>"

== system mcb_pmsm_param_est_f28379d/Parameter Estimation/Param Est/RsTest ==
  HWInputs : Inport
  StartEst : Inport  Port=2
  Config : Inport  Port=3
  Enable : EnablePort  StatesWhenEnabling=reset
  Bus Selector : BusSelector  OutputSignals=Iabc,Vdc
  Rs Estimator : mcbpmsmparamestlib/Rs Estimator
  Vabc : Outport
  Rs : Outport  Port=2
  Log : Outport  Port=3
  wires:
  Rs Estimator/1 -> Vabc/1
  HWInputs/1 -> Bus Selector/1
  Rs Estimator/2 -> Rs/1
  Rs Estimator/3 -> Log/1
  Bus Selector/1 -> Rs Estimator/1  "<Iabc>"
  Bus Selector/2 -> Rs Estimator/2  "<Vdc>"
  Config/1 -> Rs Estimator/4
  StartEst/1 -> Rs Estimator/3

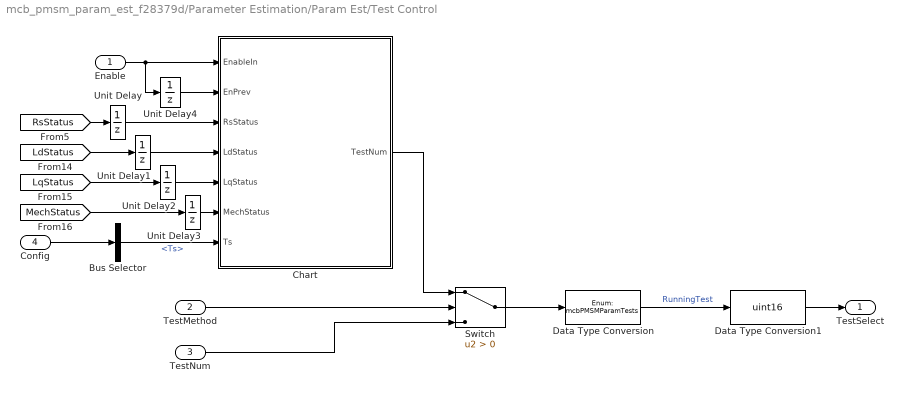
== system mcb_pmsm_param_est_f28379d/Parameter Estimation/Param Est/Test Control ==
  Enable : Inport
  TestMethod : Inport  Port=2
  TestNum : Inport  Port=3
  Config : Inport  Port=4
  Bus Selector : BusSelector  OutputSignals=Ts
  Chart : Stateflow chart  TreatAsAtomicUnit=on
  Data Type Conversion : DataTypeConversion  OutDataTypeStr=Enum: mcbPMSMParamTests  RndMeth=Simplest  SaturateOnIntegerOverflow=off
  Data Type Conversion1 : DataTypeConversion  OutDataTypeStr=uint16  RndMeth=Simplest  SaturateOnIntegerOverflow=off
  Switch : Switch  Criteria=u2 > Threshold  SaturateOnIntegerOverflow=off  InputSameDT=off
  Unit Delay{,1..4} (5 alike) : UnitDelay  SampleTime=-1  HasFrameUpgradeWarning=on
  TestSelect : Outport
  wires:
  Switch/1 -> Data Type Conversion/1
  Chart/1(TestNum) -> Switch/1
  Enable/1 -> Unit Delay4/1, Chart/1(EnableIn)
  [RsStatus] -> Unit Delay/1
  [LdStatus] -> Unit Delay1/1
  [LqStatus] -> Unit Delay2/1
  [MechStatus] -> Unit Delay3/1
  Unit Delay/1 -> Chart/3(RsStatus)
  Unit Delay1/1 -> Chart/4(LdStatus)
  Unit Delay2/1 -> Chart/5(LqStatus)
  Unit Delay3/1 -> Chart/6(MechStatus)
  Unit Delay4/1 -> Chart/2(EnPrev)
  TestMethod/1 -> Switch/2
  TestNum/1 -> Switch/3
  Data Type Conversion/1 -> Data Type Conversion1/1  "RunningTest"
  Data Type Conversion1/1 -> TestSelect/1
  Config/1 -> Bus Selector/1
  Bus Selector/1 -> Chart/7(Ts)  "<Ts>"

== system mcb_pmsm_param_est_f28379d/Parameter Estimation/Variant Subsystem/Codegen ==
  In1 : Inport
  Ground : Ground
  Terminator : Terminator
  Out1 : Outport
  wires:
  In1/1 -> Terminator/1
  Ground/1 -> Out1/1

== system mcb_pmsm_param_est_f28379d/Parameter Estimation/Variant Subsystem/Sim ==
  In1 : Inport
  Bus Selector : BusSelector  OutputSignals=Rs,Ld,Lq,Ke,B
  Mux : Mux  Inputs=5
  Out1 : Outport
  wires:
  In1/1 -> Bus Selector/1
  Bus Selector/1 -> Mux/1  "<Rs>"
  Bus Selector/2 -> Mux/2  "<Ld>"
  Bus Selector/3 -> Mux/3  "<Lq>"
  Bus Selector/4 -> Mux/4  "<Ke>"
  Bus Selector/5 -> Mux/5  "<B>"
  Mux/1 -> Out1/1

== system mcb_pmsm_param_est_f28379d/Serial Receive/Variant Subsystem/Codegen ==
  Demux : Demux  Outputs=2
  SCI Receive : c280xlib/SCI Receive  sciModule=A  dataHead=''  headerCheckMaxCount=16  dataTail=''  dataType=single  dataLenOptions=Length via dialog  dataDim=2  maxDataLength=1  initValue=0  errOption=Output the last received value  errValue=0  sampleTime=-1  blockingMode=on  timeOut=inf  outputStatus=off
  Subsystem : Subsystem
  Enable : Outport
  TestMethod : Outport  Port=2
  TestSelect : Outport  Port=3
  DebugSelect : Outport  Port=4
  Config : Outport  Port=5
  wires:
  SCI Receive/1 -> Demux/1
  Subsystem/4(TestSelect) -> TestSelect/1
  Subsystem/3(TestMethod) -> TestMethod/1
  Subsystem/2(Enable) -> Enable/1
  Demux/1 -> Subsystem/1(Count)
  Subsystem/1(Config) -> Config/1
  Demux/2 -> Subsystem/2(Data)
  Subsystem/5(DebugSelect) -> DebugSelect/1

== system mcb_pmsm_param_est_f28379d/Serial Receive/Variant Subsystem/Sim ==
  DebugDataSelect : Constant  OutDataTypeStr=uint16
  Parameter Estimation Configurator : mcbpmsmparamestlib/Parameter Estimation Configurator  P=motor.p  NRated=motor.N_rated  IRated=motor.I_rated  ImaxInverter=inverter.ISenseMax  RBoard=inverter.R_board  ISenseGain=0.0105  VSenseGain=0.0098  FreqMax=1000  FreqMin=400  FreqStepSweep=100  FreqStepEst=10  FreqNum=10  CurrMeasDelay=2 * 50e-6  KeTime=5  KeSpeed=motor.N_rated * 0.9  IqRefFOC=0.2  KpKiInputEnable=off  Kp=1  Ki=10  JSpeedLow=motor.N_rated * 0.2  DataType=single  Ts=Ts
  Test Enable : Constant  OutDataTypeStr=Inherit: Inherit via back propagation
  Test Method : Constant  OutDataTypeStr=Inherit: Inherit via back propagation
  Test Select : Constant  Value=0  OutDataTypeStr=uint16
  Enable : Outport
  TestMethod : Outport  Port=2
  TestSelect : Outport  Port=3
  DebugSelect : Outport  Port=4
  Config : Outport  Port=5
  wires:
  Test Select/1 -> TestSelect/1
  Test Method/1 -> TestMethod/1
  Test Enable/1 -> Enable/1
  Parameter Estimation Configurator/1 -> Config/1
  DebugDataSelect/1 -> DebugSelect/1

== system mcb_pmsm_param_est_f28379d/Hardware Init/Variant Subsystem/Code Generation/Calculate ADC Offset  ==
  Enable : EnablePort
  Constant : Constant  Value=8
  Constant1 : Constant  Value=inverter.CtSensOffsetMax  OutDataTypeStr=Inherit: Inherit via back propagation
  Constant2 : Constant  Value=inverter.CtSensOffsetMin  OutDataTypeStr=Inherit: Inherit via back propagation
  Divide : Product  Inputs=*/  OutDataTypeStr=uint16
  Divide1 : Product  Inputs=*/  OutDataTypeStr=uint16
  For Iterator Subsystem : Subsystem  TreatAsAtomicUnit=on
  If : If  NumInputs=3  IfExpression=u1 > u3 & u1 < u2
  If Action Subsystem : Subsystem  TreatAsAtomicUnit=on
  If Action Subsystem1 : Subsystem  TreatAsAtomicUnit=on
  If Action Subsystem2 : Subsystem  TreatAsAtomicUnit=on
  If Action Subsystem3 : Subsystem  TreatAsAtomicUnit=on
  If1 : If  NumInputs=3  IfExpression=u1 > u3 & u1 < u2
  wires:
  If1/2 -> If Action Subsystem3/Action
  If1/1 -> If Action Subsystem2/Action
  Constant1/1 -> If1/2, If/2
  If/2 -> If Action Subsystem1/Action
  For Iterator Subsystem/1(Out1) -> Divide/1
  If/1 -> If Action Subsystem/Action
  Constant2/1 -> If1/3, If/3
  For Iterator Subsystem/2(Out2) -> Divide1/1
  Divide1/1 -> If1/1, If Action Subsystem2/1(In1)
  Constant/1 -> Divide1/2, Divide/2
  Divide/1 -> If Action Subsystem/1(In1), If/1

== system mcb_pmsm_param_est_f28379d/Hardware Init/Variant Subsystem/Code Generation/DRV Enable ==
  note: Enable inverter
  In : Inport
  ADC Gain setting : Subsystem
  Constant : Constant  Value=inverter.EnableLogic
  Digital Output : c2837xDlib/Digital Output  Priority=10  GPIO_Number=GPIO120~GPIO127  GPIO_Bit0=off  GPIO_BIT0_Toggle=off  GPIO_Bit1=off  GPIO_BIT1_Toggle=off  GPIO_Bit2=off  GPIO_BIT2_Toggle=off  GPIO_Bit3=off  GPIO_BIT3_Toggle=off  GPIO_Bit4=on  GPIO_BIT4_Toggle=off  GPIO_Bit5=off  GPIO_BIT5_Toggle=off  GPIO_Bit6=off  GPIO_BIT6_Toggle=off  GPIO_Bit7=off  GPIO_BIT7_Toggle=off
  Digital Output1 : c2837xDlib/Digital Output  Priority=10  GPIO_Number=GPIO16~GPIO23  GPIO_Bit0=off  GPIO_BIT0_Toggle=off  GPIO_Bit1=off  GPIO_BIT1_Toggle=off  GPIO_Bit2=off  GPIO_BIT2_Toggle=off  GPIO_Bit3=off  GPIO_BIT3_Toggle=off  GPIO_Bit4=off  GPIO_BIT4_Toggle=off  GPIO_Bit5=off  GPIO_BIT5_Toggle=off  GPIO_Bit6=on  GPIO_BIT6_Toggle=off  GPIO_Bit7=off  GPIO_BIT7_Toggle=off
  Inverter Enable : Constant  OutDataTypeStr=uint16  SampleTime=-1
  NOT : Logic  Operator=NOT  IconShape=distinctive  AllPortsSameDT=off  OutDataTypeStr=boolean
  RunTimeMeasurement : Constant  OutDataTypeStr=uint16  SampleTime=-1
  Switch : Switch  Criteria=u2 > Threshold  SaturateOnIntegerOverflow=off  InputSameDT=off
  wires:
  Inverter Enable/1 -> Switch/1, NOT/1  "Active high logic for inverter enable"
  RunTimeMeasurement/1 -> Digital Output1/1
  Constant/1 -> ADC Gain setting/Enable, Switch/2
  Switch/1 -> Digital Output/1
  NOT/1 -> Switch/3  "Active low logic for inverter enable"
  In/1 -> ADC Gain setting/1(In1)

== system mcb_pmsm_param_est_f28379d/Hardware Init/Variant Subsystem/Code Generation/Default ADC Offset ==
  Enable : EnablePort
  Constant : Constant  Value=inverter.CtSensAOffset  OutDataTypeStr=Inherit: Inherit via back propagation
  Constant1 : Constant  Value=inverter.CtSensBOffset  OutDataTypeStr=Inherit: Inherit via back propagation
  Data Store Write1 : DataStoreWrite  DataStoreName=IaOffset  IndexOptions=Index vector (dialog)  Indices=1  OutputSizes=1
  Data Store Write2 : DataStoreWrite  DataStoreName=IbOffset  IndexOptions=Index vector (dialog)  Indices=1  OutputSizes=1
  wires:
  Constant/1 -> Data Store Write1/1
  Constant1/1 -> Data Store Write2/1

== system mcb_pmsm_param_est_f28379d/Inverter and Motor/Inverter and Motor/Sim/Inverter ==
  Duty_abc : Inport
  Average-Value Inverter : mcbplantlib/Average-Value Inverter
  Constant2 : Constant  Value=inverter.V_dc  OutDataTypeStr=single  SampleTime=-1
  Data Type Conversion1 : DataTypeConversion  OutDataTypeStr=single  RndMeth=Simplest  SaturateOnIntegerOverflow=off
  Rate Transition3 : RateTransition  Deterministic=off  OutPortSampleTime=Ts_inverter
  Vabc : Outport  VectorParamsAs1DForOutWhenUnconnected=off
  wires:
  Constant2/1 -> Average-Value Inverter/2
  Data Type Conversion1/1 -> Rate Transition3/1
  Duty_abc/1 -> Data Type Conversion1/1
  Rate Transition3/1 -> Average-Value Inverter/1
  Average-Value Inverter/1 -> Vabc/1

== system mcb_pmsm_param_est_f28379d/Inverter and Motor/Inverter and Motor/Sim/Motor ==
  note: Note :
      | The PMSM block does not simulate magentic effects of the rotor when Vd is applied. In order to simulate locking of the rotor at zero position, PMSM block is used in zero speed input during Rs, Ld and Lq estimation.
      | Do not use simulation to determine the Vd value required to align the rotor at zero position.
  PhaseVolt : Inport
  ActiveTest : Inport  Port=2
  ActiveTest1 : InportShadow  Port=2
  Constant : Constant  Value=0  OutDataTypeStr=single
  Constant1 : Constant  Value=0  OutDataTypeStr=single
  "Interior PMSM with free rotor (Ke, J, B)" : autolibpmsminterior/Interior PMSM  port_config=Torque  sim_type=Discrete  Ts=Ts_motor  P=motor.p  Rs=motor.Rs +inverter.R_board  Ldq=[motor.Ld motor.Lq]  KConstText=Permanent flux linkage constant (lambda_pm):  lambda_pm=motor.FluxPM  Ke=159.9771  mechanical=[motor.J, motor.B, 0]  idq0=[0 0]  theta_init=0  omega_init=0  KConst=motor.FluxPM  lambda_pm_calc=motor.FluxPM  Kt=0.07  RefBlkName='autolibpmsminterior/Interior PMSM'  aMode=5
      settings: LibrarySourceBlock=mcblib/Electrical Systems/Motors/Interior PMSM
  "Interior PMSM with locked rotor (Rs, Ld, Lq)" : autolibpmsminterior/Interior PMSM  port_config=Speed  sim_type=Discrete  Ts=Ts_motor  P=motor.p  Rs=motor.Rs +inverter.R_board  Ldq=[motor.Ld motor.Lq]  KConstText=Permanent flux linkage constant (lambda_pm):  lambda_pm=motor.FluxPM  Ke=159.9771  mechanical=[motor.J, motor.B, 0]  idq0=[0 0]  theta_init=0  omega_init=0  KConst=motor.FluxPM  lambda_pm_calc=motor.FluxPM  Kt=0.07  RefBlkName='autolibpmsminterior/Interior PMSM'  aMode=5
      settings: LibrarySourceBlock=mcblib/Electrical Systems/Motors/Interior PMSM
  PhaseVolt1 : InportShadow
  Switch : Switch  Criteria=u2 > Threshold  Threshold=3  SaturateOnIntegerOverflow=off  InputSameDT=off
  Switch1 : Switch  Criteria=u2 > Threshold  Threshold=3  SaturateOnIntegerOverflow=off  InputSameDT=off
  Terminator : Terminator
  Terminator1 : Terminator
  Info : Outport
  Iabc : Outport  Port=2
  wires:
  PhaseVolt/1 -> "Interior PMSM with free rotor (Ke, J, B)"/2
  Constant/1 -> "Interior PMSM with free rotor (Ke, J, B)"/1
  PhaseVolt1/1 -> "Interior PMSM with locked rotor (Rs, Ld, Lq)"/2
  Constant1/1 -> "Interior PMSM with locked rotor (Rs, Ld, Lq)"/1
  "Interior PMSM with free rotor (Ke, J, B)"/3 -> Terminator/1
  "Interior PMSM with locked rotor (Rs, Ld, Lq)"/3 -> Terminator1/1
  Switch/1 -> Info/1
  ActiveTest/1 -> Switch/2
  "Interior PMSM with free rotor (Ke, J, B)"/1 -> Switch/1
  Switch1/1 -> Iabc/1
  ActiveTest1/1 -> Switch1/2
  "Interior PMSM with locked rotor (Rs, Ld, Lq)"/1 -> Switch/3
  "Interior PMSM with free rotor (Ke, J, B)"/2 -> Switch1/1  "Iabc"
  "Interior PMSM with locked rotor (Rs, Ld, Lq)"/2 -> Switch1/3  "Iabc"
